simulink model "PSB3_0"  (R2021a)
settings: Solver=VariableStepAuto  StartTime=0.0  StopTime=3000  RelTol=1e-3
values from neighbouring files (symbols this model uses):
  n_channel = 1024    [PSB3_0_script.m]    (also in PSB_FPGAdesign8_script.m)
  parallel_factor = 4    [PSB3_0_script.m]    (also in PSB_FPGAdesign8_script.m)
libraries: xbsIndex_r4 x1051, xrbsSSR_Library x154, dspsrcs4 x26
(part 4 of 8)

== system PSB3_0/Overflow Detector add_re_1 ==
  rst : Inport
  A : Inport  Port=2
  B : Inport  Port=3
  S : Inport  Port=4
  Constant17 : xbsIndex_r4/Constant  const=1  gui_display_data_type=Boolean  arith_type=Boolean  n_bits=16  bin_pt=14  preci_type=Single  exp_width=8  frac_width=24  explicit_period=on  period=1  equ=P=C  opselect=C  inp2=PCIN>>17  opr=+  inp1=P  carry=CIN  dbl_ovrd=off  block_type=constant
  Convert : xbsIndex_r4/Convert  gui_display_data_type=Boolean  arith_type=Boolean  n_bits=16  bin_pt=14  float_type=Single  exp_bits=8  fraction_bits=24  quantization=Truncate  overflow=Wrap  en=off  latency=1  pipeline=off  dbl_ovrd=off  block_type=convert
  Expression : xbsIndex_r4/Expression  expression=(A & B & ~S) | (~A & ~B & S)  align_bp=off  en=off  latency=1  precision=User Defined  arith_type=Unsigned  n_bits=1  bin_pt=0  dbl_ovrd=off  block_type=expr
  Register : xbsIndex_r4/Register  init=0  rst=on  en=on  dbl_ovrd=off  block_type=register
  Vector Delay : xrbsSSR_Library/Vector Delay  sg_latency=2  infoeditControl=Selection of Reset will increase slice count due to use of real FFs and instead of SRLs  en=off  vectorize_en=off  rst=off  reg_retiming=off  block_type=delay_ssr  dbl_ovrd=off  sg_ssr=16  sg_ssr_prev=16  sg_ssr_name=vect_delay
      settings: SourceProductName=Xilinx SSR Blockset
  Vector Delay1 : xrbsSSR_Library/Vector Delay  sg_latency=2  infoeditControl=Selection of Reset will increase slice count due to use of real FFs and instead of SRLs  en=off  vectorize_en=off  rst=off  reg_retiming=off  block_type=delay_ssr  dbl_ovrd=off  sg_ssr=16  sg_ssr_prev=16  sg_ssr_name=vect_delay
      settings: SourceProductName=Xilinx SSR Blockset
  Vector Slice : xrbsSSR_Library/Vector Slice  nbits=1  sg_ssr=16  sg_ssr_prev=16  boolean_output=on  mode=Upper Bit Location + Width  bit1=0  base1=MSB of Input  bit0=0  base0=LSB of Input  dbl_ovrd=off  block_type=slice_ssr  sg_ssr_name=vect_slice
      settings: SourceProductName=Xilinx SSR Blockset  infoedit="The Vector Slice block supports input of vector types. Extracts a given range of bits from each sample of input vector and presents it at the output.  The output type is ordinarily unsigned with binary point at zero, but can be Boolean when the slice is one bit wide.<br><br>Hardware notes: In hardware this block costs nothing."
  Vector Slice1 : xrbsSSR_Library/Vector Slice  nbits=1  sg_ssr=16  sg_ssr_prev=16  boolean_output=on  mode=Upper Bit Location + Width  bit1=0  base1=MSB of Input  bit0=0  base0=LSB of Input  dbl_ovrd=off  block_type=slice_ssr  sg_ssr_name=vect_slice
      settings: SourceProductName=Xilinx SSR Blockset  infoedit="The Vector Slice block supports input of vector types. Extracts a given range of bits from each sample of input vector and presents it at the output.  The output type is ordinarily unsigned with binary point at zero, but can be Boolean when the slice is one bit wide.<br><br>Hardware notes: In hardware this block costs nothing."
  Vector Slice2 : xrbsSSR_Library/Vector Slice  nbits=1  sg_ssr=16  sg_ssr_prev=16  boolean_output=on  mode=Upper Bit Location + Width  bit1=0  base1=MSB of Input  bit0=0  base0=LSB of Input  dbl_ovrd=off  block_type=slice_ssr  sg_ssr_name=vect_slice
      settings: SourceProductName=Xilinx SSR Blockset  infoedit="The Vector Slice block supports input of vector types. Extracts a given range of bits from each sample of input vector and presents it at the output.  The output type is ordinarily unsigned with binary point at zero, but can be Boolean when the slice is one bit wide.<br><br>Hardware notes: In hardware this block costs nothing."
  Vector to Scalar : xrbsSSR_Library/Vector2Scalar  sg_ssr=16  sg_ssr_prev=16  sg_ssr_name=vect_Vector2Scalar  block_type=vector2scalar_ssr
      settings: SourceProductName=Xilinx SSR Blockset
  Vector to Scalar1 : xrbsSSR_Library/Vector2Scalar  sg_ssr=16  sg_ssr_prev=16  sg_ssr_name=vect_Vector2Scalar  block_type=vector2scalar_ssr
      settings: SourceProductName=Xilinx SSR Blockset
  Vector to Scalar2 : xrbsSSR_Library/Vector2Scalar  sg_ssr=16  sg_ssr_prev=16  sg_ssr_name=vect_Vector2Scalar  block_type=vector2scalar_ssr
      settings: SourceProductName=Xilinx SSR Blockset
  ov : Outport
  wires:
  Register/1 -> ov/1
  A/1 -> Vector Slice/1
  rst/1 -> Register/2
  Constant17/1 -> Register/1
  B/1 -> Vector Slice1/1
  S/1 -> Vector Slice2/1
  Vector Slice/1 -> Vector Delay/1
  Vector Slice1/1 -> Vector Delay1/1
  Vector Delay/1 -> Vector to Scalar/1
  Vector Delay1/1 -> Vector to Scalar1/1
  Vector Slice2/1 -> Vector to Scalar2/1
  Vector to Scalar/1 -> Expression/1
  Vector to Scalar1/1 -> Expression/2
  Vector to Scalar2/1 -> Expression/3
  Expression/1 -> Convert/1
  Convert/1 -> Register/3

== system PSB3_0/Overflow Detector add_re_2 ==
  rst : Inport
  A : Inport  Port=2
  B : Inport  Port=3
  S : Inport  Port=4
  Constant17 : xbsIndex_r4/Constant  const=1  gui_display_data_type=Boolean  arith_type=Boolean  n_bits=16  bin_pt=14  preci_type=Single  exp_width=8  frac_width=24  explicit_period=on  period=1  equ=P=C  opselect=C  inp2=PCIN>>17  opr=+  inp1=P  carry=CIN  dbl_ovrd=off  block_type=constant
  Convert : xbsIndex_r4/Convert  gui_display_data_type=Boolean  arith_type=Boolean  n_bits=16  bin_pt=14  float_type=Single  exp_bits=8  fraction_bits=24  quantization=Truncate  overflow=Wrap  en=off  latency=1  pipeline=off  dbl_ovrd=off  block_type=convert
  Expression : xbsIndex_r4/Expression  expression=(A & B & ~S) | (~A & ~B & S)  align_bp=off  en=off  latency=1  precision=User Defined  arith_type=Unsigned  n_bits=1  bin_pt=0  dbl_ovrd=off  block_type=expr
  Register : xbsIndex_r4/Register  init=0  rst=on  en=on  dbl_ovrd=off  block_type=register
  Vector Delay : xrbsSSR_Library/Vector Delay  sg_latency=2  infoeditControl=Selection of Reset will increase slice count due to use of real FFs and instead of SRLs  en=off  vectorize_en=off  rst=off  reg_retiming=off  block_type=delay_ssr  dbl_ovrd=off  sg_ssr=16  sg_ssr_prev=16  sg_ssr_name=vect_delay
      settings: SourceProductName=Xilinx SSR Blockset
  Vector Delay1 : xrbsSSR_Library/Vector Delay  sg_latency=2  infoeditControl=Selection of Reset will increase slice count due to use of real FFs and instead of SRLs  en=off  vectorize_en=off  rst=off  reg_retiming=off  block_type=delay_ssr  dbl_ovrd=off  sg_ssr=16  sg_ssr_prev=16  sg_ssr_name=vect_delay
      settings: SourceProductName=Xilinx SSR Blockset
  Vector Slice : xrbsSSR_Library/Vector Slice  nbits=1  sg_ssr=16  sg_ssr_prev=16  boolean_output=on  mode=Upper Bit Location + Width  bit1=0  base1=MSB of Input  bit0=0  base0=LSB of Input  dbl_ovrd=off  block_type=slice_ssr  sg_ssr_name=vect_slice
      settings: SourceProductName=Xilinx SSR Blockset  infoedit="The Vector Slice block supports input of vector types. Extracts a given range of bits from each sample of input vector and presents it at the output.  The output type is ordinarily unsigned with binary point at zero, but can be Boolean when the slice is one bit wide.<br><br>Hardware notes: In hardware this block costs nothing."
  Vector Slice1 : xrbsSSR_Library/Vector Slice  nbits=1  sg_ssr=16  sg_ssr_prev=16  boolean_output=on  mode=Upper Bit Location + Width  bit1=0  base1=MSB of Input  bit0=0  base0=LSB of Input  dbl_ovrd=off  block_type=slice_ssr  sg_ssr_name=vect_slice
      settings: SourceProductName=Xilinx SSR Blockset  infoedit="The Vector Slice block supports input of vector types. Extracts a given range of bits from each sample of input vector and presents it at the output.  The output type is ordinarily unsigned with binary point at zero, but can be Boolean when the slice is one bit wide.<br><br>Hardware notes: In hardware this block costs nothing."
  Vector Slice2 : xrbsSSR_Library/Vector Slice  nbits=1  sg_ssr=16  sg_ssr_prev=16  boolean_output=on  mode=Upper Bit Location + Width  bit1=0  base1=MSB of Input  bit0=0  base0=LSB of Input  dbl_ovrd=off  block_type=slice_ssr  sg_ssr_name=vect_slice
      settings: SourceProductName=Xilinx SSR Blockset  infoedit="The Vector Slice block supports input of vector types. Extracts a given range of bits from each sample of input vector and presents it at the output.  The output type is ordinarily unsigned with binary point at zero, but can be Boolean when the slice is one bit wide.<br><br>Hardware notes: In hardware this block costs nothing."
  Vector to Scalar : xrbsSSR_Library/Vector2Scalar  sg_ssr=16  sg_ssr_prev=16  sg_ssr_name=vect_Vector2Scalar  block_type=vector2scalar_ssr
      settings: SourceProductName=Xilinx SSR Blockset
  Vector to Scalar1 : xrbsSSR_Library/Vector2Scalar  sg_ssr=16  sg_ssr_prev=16  sg_ssr_name=vect_Vector2Scalar  block_type=vector2scalar_ssr
      settings: SourceProductName=Xilinx SSR Blockset
  Vector to Scalar2 : xrbsSSR_Library/Vector2Scalar  sg_ssr=16  sg_ssr_prev=16  sg_ssr_name=vect_Vector2Scalar  block_type=vector2scalar_ssr
      settings: SourceProductName=Xilinx SSR Blockset
  ov : Outport
  wires:
  Register/1 -> ov/1
  A/1 -> Vector Slice/1
  rst/1 -> Register/2
  Constant17/1 -> Register/1
  B/1 -> Vector Slice1/1
  S/1 -> Vector Slice2/1
  Vector Slice/1 -> Vector Delay/1
  Vector Slice1/1 -> Vector Delay1/1
  Vector Delay/1 -> Vector to Scalar/1
  Vector Delay1/1 -> Vector to Scalar1/1
  Vector Slice2/1 -> Vector to Scalar2/1
  Vector to Scalar/1 -> Expression/1
  Vector to Scalar1/1 -> Expression/2
  Vector to Scalar2/1 -> Expression/3
  Expression/1 -> Convert/1
  Convert/1 -> Register/3

== system PSB3_0/Overflow Detector add_re_3 ==
  rst : Inport
  A : Inport  Port=2
  B : Inport  Port=3
  S : Inport  Port=4
  Constant17 : xbsIndex_r4/Constant  const=1  gui_display_data_type=Boolean  arith_type=Boolean  n_bits=16  bin_pt=14  preci_type=Single  exp_width=8  frac_width=24  explicit_period=on  period=1  equ=P=C  opselect=C  inp2=PCIN>>17  opr=+  inp1=P  carry=CIN  dbl_ovrd=off  block_type=constant
  Convert : xbsIndex_r4/Convert  gui_display_data_type=Boolean  arith_type=Boolean  n_bits=16  bin_pt=14  float_type=Single  exp_bits=8  fraction_bits=24  quantization=Truncate  overflow=Wrap  en=off  latency=1  pipeline=off  dbl_ovrd=off  block_type=convert
  Expression : xbsIndex_r4/Expression  expression=(A & B & ~S) | (~A & ~B & S)  align_bp=off  en=off  latency=1  precision=User Defined  arith_type=Unsigned  n_bits=1  bin_pt=0  dbl_ovrd=off  block_type=expr
  Register : xbsIndex_r4/Register  init=0  rst=on  en=on  dbl_ovrd=off  block_type=register
  Vector Delay : xrbsSSR_Library/Vector Delay  sg_latency=2  infoeditControl=Selection of Reset will increase slice count due to use of real FFs and instead of SRLs  en=off  vectorize_en=off  rst=off  reg_retiming=off  block_type=delay_ssr  dbl_ovrd=off  sg_ssr=16  sg_ssr_prev=16  sg_ssr_name=vect_delay
      settings: SourceProductName=Xilinx SSR Blockset
  Vector Delay1 : xrbsSSR_Library/Vector Delay  sg_latency=2  infoeditControl=Selection of Reset will increase slice count due to use of real FFs and instead of SRLs  en=off  vectorize_en=off  rst=off  reg_retiming=off  block_type=delay_ssr  dbl_ovrd=off  sg_ssr=16  sg_ssr_prev=16  sg_ssr_name=vect_delay
      settings: SourceProductName=Xilinx SSR Blockset
  Vector Slice : xrbsSSR_Library/Vector Slice  nbits=1  sg_ssr=16  sg_ssr_prev=16  boolean_output=on  mode=Upper Bit Location + Width  bit1=0  base1=MSB of Input  bit0=0  base0=LSB of Input  dbl_ovrd=off  block_type=slice_ssr  sg_ssr_name=vect_slice
      settings: SourceProductName=Xilinx SSR Blockset  infoedit="The Vector Slice block supports input of vector types. Extracts a given range of bits from each sample of input vector and presents it at the output.  The output type is ordinarily unsigned with binary point at zero, but can be Boolean when the slice is one bit wide.<br><br>Hardware notes: In hardware this block costs nothing."
  Vector Slice1 : xrbsSSR_Library/Vector Slice  nbits=1  sg_ssr=16  sg_ssr_prev=16  boolean_output=on  mode=Upper Bit Location + Width  bit1=0  base1=MSB of Input  bit0=0  base0=LSB of Input  dbl_ovrd=off  block_type=slice_ssr  sg_ssr_name=vect_slice
      settings: SourceProductName=Xilinx SSR Blockset  infoedit="The Vector Slice block supports input of vector types. Extracts a given range of bits from each sample of input vector and presents it at the output.  The output type is ordinarily unsigned with binary point at zero, but can be Boolean when the slice is one bit wide.<br><br>Hardware notes: In hardware this block costs nothing."
  Vector Slice2 : xrbsSSR_Library/Vector Slice  nbits=1  sg_ssr=16  sg_ssr_prev=16  boolean_output=on  mode=Upper Bit Location + Width  bit1=0  base1=MSB of Input  bit0=0  base0=LSB of Input  dbl_ovrd=off  block_type=slice_ssr  sg_ssr_name=vect_slice
      settings: SourceProductName=Xilinx SSR Blockset  infoedit="The Vector Slice block supports input of vector types. Extracts a given range of bits from each sample of input vector and presents it at the output.  The output type is ordinarily unsigned with binary point at zero, but can be Boolean when the slice is one bit wide.<br><br>Hardware notes: In hardware this block costs nothing."
  Vector to Scalar : xrbsSSR_Library/Vector2Scalar  sg_ssr=16  sg_ssr_prev=16  sg_ssr_name=vect_Vector2Scalar  block_type=vector2scalar_ssr
      settings: SourceProductName=Xilinx SSR Blockset
  Vector to Scalar1 : xrbsSSR_Library/Vector2Scalar  sg_ssr=16  sg_ssr_prev=16  sg_ssr_name=vect_Vector2Scalar  block_type=vector2scalar_ssr
      settings: SourceProductName=Xilinx SSR Blockset
  Vector to Scalar2 : xrbsSSR_Library/Vector2Scalar  sg_ssr=16  sg_ssr_prev=16  sg_ssr_name=vect_Vector2Scalar  block_type=vector2scalar_ssr
      settings: SourceProductName=Xilinx SSR Blockset
  ov : Outport
  wires:
  Register/1 -> ov/1
  A/1 -> Vector Slice/1
  rst/1 -> Register/2
  Constant17/1 -> Register/1
  B/1 -> Vector Slice1/1
  S/1 -> Vector Slice2/1
  Vector Slice/1 -> Vector Delay/1
  Vector Slice1/1 -> Vector Delay1/1
  Vector Delay/1 -> Vector to Scalar/1
  Vector Delay1/1 -> Vector to Scalar1/1
  Vector Slice2/1 -> Vector to Scalar2/1
  Vector to Scalar/1 -> Expression/1
  Vector to Scalar1/1 -> Expression/2
  Vector to Scalar2/1 -> Expression/3
  Expression/1 -> Convert/1
  Convert/1 -> Register/3

== system PSB3_0/Overflow Detector add_re_4 ==
  rst : Inport
  A : Inport  Port=2
  B : Inport  Port=3
  S : Inport  Port=4
  Constant17 : xbsIndex_r4/Constant  const=1  gui_display_data_type=Boolean  arith_type=Boolean  n_bits=16  bin_pt=14  preci_type=Single  exp_width=8  frac_width=24  explicit_period=on  period=1  equ=P=C  opselect=C  inp2=PCIN>>17  opr=+  inp1=P  carry=CIN  dbl_ovrd=off  block_type=constant
  Convert : xbsIndex_r4/Convert  gui_display_data_type=Boolean  arith_type=Boolean  n_bits=16  bin_pt=14  float_type=Single  exp_bits=8  fraction_bits=24  quantization=Truncate  overflow=Wrap  en=off  latency=1  pipeline=off  dbl_ovrd=off  block_type=convert
  Expression : xbsIndex_r4/Expression  expression=(A & B & ~S) | (~A & ~B & S)  align_bp=off  en=off  latency=1  precision=User Defined  arith_type=Unsigned  n_bits=1  bin_pt=0  dbl_ovrd=off  block_type=expr
  Register : xbsIndex_r4/Register  init=0  rst=on  en=on  dbl_ovrd=off  block_type=register
  Vector Delay : xrbsSSR_Library/Vector Delay  sg_latency=2  infoeditControl=Selection of Reset will increase slice count due to use of real FFs and instead of SRLs  en=off  vectorize_en=off  rst=off  reg_retiming=off  block_type=delay_ssr  dbl_ovrd=off  sg_ssr=16  sg_ssr_prev=16  sg_ssr_name=vect_delay
      settings: SourceProductName=Xilinx SSR Blockset
  Vector Delay1 : xrbsSSR_Library/Vector Delay  sg_latency=2  infoeditControl=Selection of Reset will increase slice count due to use of real FFs and instead of SRLs  en=off  vectorize_en=off  rst=off  reg_retiming=off  block_type=delay_ssr  dbl_ovrd=off  sg_ssr=16  sg_ssr_prev=16  sg_ssr_name=vect_delay
      settings: SourceProductName=Xilinx SSR Blockset
  Vector Slice : xrbsSSR_Library/Vector Slice  nbits=1  sg_ssr=16  sg_ssr_prev=16  boolean_output=on  mode=Upper Bit Location + Width  bit1=0  base1=MSB of Input  bit0=0  base0=LSB of Input  dbl_ovrd=off  block_type=slice_ssr  sg_ssr_name=vect_slice
      settings: SourceProductName=Xilinx SSR Blockset  infoedit="The Vector Slice block supports input of vector types. Extracts a given range of bits from each sample of input vector and presents it at the output.  The output type is ordinarily unsigned with binary point at zero, but can be Boolean when the slice is one bit wide.<br><br>Hardware notes: In hardware this block costs nothing."
  Vector Slice1 : xrbsSSR_Library/Vector Slice  nbits=1  sg_ssr=16  sg_ssr_prev=16  boolean_output=on  mode=Upper Bit Location + Width  bit1=0  base1=MSB of Input  bit0=0  base0=LSB of Input  dbl_ovrd=off  block_type=slice_ssr  sg_ssr_name=vect_slice
      settings: SourceProductName=Xilinx SSR Blockset  infoedit="The Vector Slice block supports input of vector types. Extracts a given range of bits from each sample of input vector and presents it at the output.  The output type is ordinarily unsigned with binary point at zero, but can be Boolean when the slice is one bit wide.<br><br>Hardware notes: In hardware this block costs nothing."
  Vector Slice2 : xrbsSSR_Library/Vector Slice  nbits=1  sg_ssr=16  sg_ssr_prev=16  boolean_output=on  mode=Upper Bit Location + Width  bit1=0  base1=MSB of Input  bit0=0  base0=LSB of Input  dbl_ovrd=off  block_type=slice_ssr  sg_ssr_name=vect_slice
      settings: SourceProductName=Xilinx SSR Blockset  infoedit="The Vector Slice block supports input of vector types. Extracts a given range of bits from each sample of input vector and presents it at the output.  The output type is ordinarily unsigned with binary point at zero, but can be Boolean when the slice is one bit wide.<br><br>Hardware notes: In hardware this block costs nothing."
  Vector to Scalar : xrbsSSR_Library/Vector2Scalar  sg_ssr=16  sg_ssr_prev=16  sg_ssr_name=vect_Vector2Scalar  block_type=vector2scalar_ssr
      settings: SourceProductName=Xilinx SSR Blockset
  Vector to Scalar1 : xrbsSSR_Library/Vector2Scalar  sg_ssr=16  sg_ssr_prev=16  sg_ssr_name=vect_Vector2Scalar  block_type=vector2scalar_ssr
      settings: SourceProductName=Xilinx SSR Blockset
  Vector to Scalar2 : xrbsSSR_Library/Vector2Scalar  sg_ssr=16  sg_ssr_prev=16  sg_ssr_name=vect_Vector2Scalar  block_type=vector2scalar_ssr
      settings: SourceProductName=Xilinx SSR Blockset
  ov : Outport
  wires:
  Register/1 -> ov/1
  A/1 -> Vector Slice/1
  rst/1 -> Register/2
  Constant17/1 -> Register/1
  B/1 -> Vector Slice1/1
  S/1 -> Vector Slice2/1
  Vector Slice/1 -> Vector Delay/1
  Vector Slice1/1 -> Vector Delay1/1
  Vector Delay/1 -> Vector to Scalar/1
  Vector Delay1/1 -> Vector to Scalar1/1
  Vector Slice2/1 -> Vector to Scalar2/1
  Vector to Scalar/1 -> Expression/1
  Vector to Scalar1/1 -> Expression/2
  Vector to Scalar2/1 -> Expression/3
  Expression/1 -> Convert/1
  Convert/1 -> Register/3

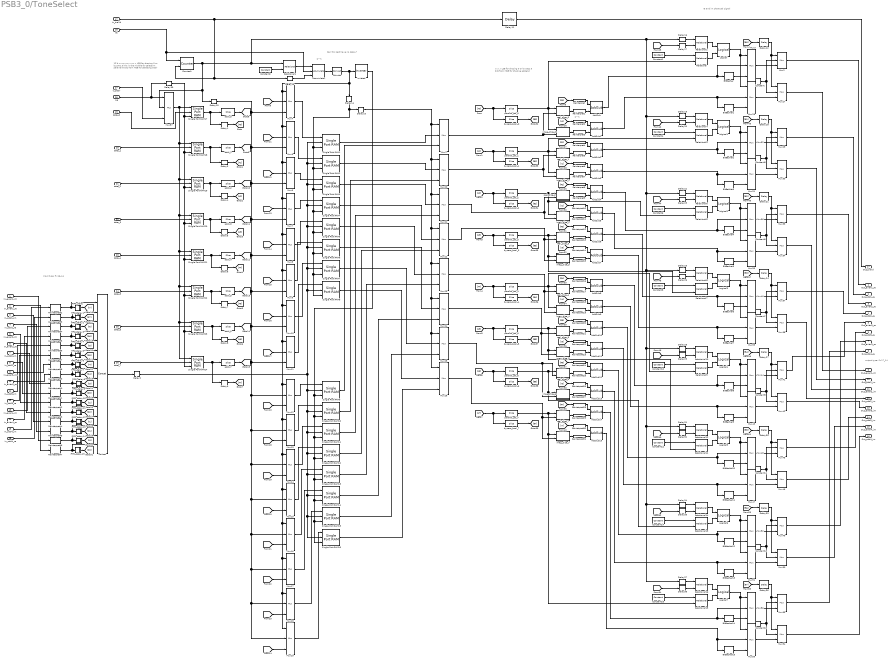
== system PSB3_0/ToneSelect ==
  note: Can this cast have no delay?
  note: Z^-1
  note: input type: fix16_14
  note: output type: fix17_14
  note: xxx,x
      | LSB for chosing 0 or bypass
      | 3 bits from MSB for chosing addend
  note: re and im share sel signal
  note: Z^-1
  note: 12'b xxxxxxxx,xxx,x
      | LSB for chosing 0 or bypass
      | 3 bits in the middle for selecting parallel
      | 8 bits from MSB for selecting addr
  In_even1_im : Inport
  In_even1_re : Inport  Port=2
  In_odd1_im : Inport  Port=3
  In_odd1_re : Inport  Port=4
  In_even2_im : Inport  Port=5
  In_even2_re : Inport  Port=6
  In_odd2_im : Inport  Port=7
  In_odd2_re : Inport  Port=8
  In_even3_im : Inport  Port=9
  In_even3_re : Inport  Port=10
  In_odd3_im : Inport  Port=11
  In_odd3_re : Inport  Port=12
  In_even4_im : Inport  Port=13
  In_even4_re : Inport  Port=14
  In_odd4_im : Inport  Port=15
  In_odd4_re : Inport  Port=16
  In_tvalid : Inport  Port=17
  rst : Inport  Port=18
  data_0 : Inport  Port=19
  data_1 : Inport  Port=20
  data_2 : Inport  Port=21
  data_3 : Inport  Port=22
  data_4 : Inport  Port=23
  data_5 : Inport  Port=24
  data_6 : Inport  Port=25
  data_7 : Inport  Port=26
  w_addr : Inport  Port=27
  we : Inport  Port=28
  Accumulator : xbsIndex_r4/Accumulator  operation=Add  n_bits=1  overflow=Wrap  scale=1  rst=on  hasbypass=off  infoeditControl=reset for floating point data type must be asserted for a minimum of 2 cycles  en=on  latency=1  msb_inp=1  msb=1  lsb=1  use_behavioral_HDL=on  implementation=Fabric  dbl_ovrd=off  block_type=accum
  AddSub{,1..15} (16 alike) : xbsIndex_r4/AddSub  mode=Addition  use_carryin=off  use_carryout=off  en=off  latency=2  precision=User Defined  arith_type="Signed  (2's comp)"  n_bits=17  bin_pt=14  quantization=Truncate  overflow=Flag as error  use_behavioral_HDL=off  hw_selection=Fabric  pipelined=off  dbl_ovrd=off  block_type=addsub
  BitBasher{,1..15} (16 alike) : xbsIndex_r4/BitBasher  bitexpr=o={i[16],i[16:1]}  display_expr=off  sr_1=o  arith_type1="Signed  (2's comp)"  bin_pt1=14  sr_2=2  arith_type2=Unsigned  bin_pt2=0  sr_3=3  arith_type3=Unsigned  bin_pt3=0  sr_4=4  arith_type4=Unsigned  bin_pt4=0  dbl_ovrd=off  block_type=bitbasher
  Concat : xbsIndex_r4/Concat  num_inputs=16  dbl_ovrd=off  block_type=concat
  Constant{,3,5,7,9,11,13,15} (8 alike) : xbsIndex_r4/Constant  const=0  gui_display_data_type=Fixed-point  arith_type=Signed (2's comp)  n_bits=17  bin_pt=14  preci_type=Single  exp_width=8  frac_width=24  explicit_period=on  period=1  equ=P=C  opselect=C  inp2=PCIN>>17  opr=+  inp1=P  carry=CIN  dbl_ovrd=off  block_type=constant
  Constant1 : xbsIndex_r4/Constant  const=0  gui_display_data_type=Fixed-point  arith_type=Unsigned  n_bits=3  bin_pt=0  preci_type=Single  exp_width=8  frac_width=24  explicit_period=on  period=1  equ=P=C  opselect=C  inp2=PCIN>>17  opr=+  inp1=P  carry=CIN  dbl_ovrd=off  block_type=constant
  Constant10 : xbsIndex_r4/Constant  const=4  gui_display_data_type=Fixed-point  arith_type=Unsigned  n_bits=3  bin_pt=0  preci_type=Single  exp_width=8  frac_width=24  explicit_period=on  period=1  equ=P=C  opselect=C  inp2=PCIN>>17  opr=+  inp1=P  carry=CIN  dbl_ovrd=off  block_type=constant
  Constant12 : xbsIndex_r4/Constant  const=5  gui_display_data_type=Fixed-point  arith_type=Unsigned  n_bits=3  bin_pt=0  preci_type=Single  exp_width=8  frac_width=24  explicit_period=on  period=1  equ=P=C  opselect=C  inp2=PCIN>>17  opr=+  inp1=P  carry=CIN  dbl_ovrd=off  block_type=constant
  Constant14 : xbsIndex_r4/Constant  const=6  gui_display_data_type=Fixed-point  arith_type=Unsigned  n_bits=3  bin_pt=0  preci_type=Single  exp_width=8  frac_width=24  explicit_period=on  period=1  equ=P=C  opselect=C  inp2=PCIN>>17  opr=+  inp1=P  carry=CIN  dbl_ovrd=off  block_type=constant
  Constant16 : xbsIndex_r4/Constant  const=7  gui_display_data_type=Fixed-point  arith_type=Unsigned  n_bits=3  bin_pt=0  preci_type=Single  exp_width=8  frac_width=24  explicit_period=on  period=1  equ=P=C  opselect=C  inp2=PCIN>>17  opr=+  inp1=P  carry=CIN  dbl_ovrd=off  block_type=constant
  Constant2 : xbsIndex_r4/Constant  const=0  gui_display_data_type=Fixed-point  arith_type=Unsigned  n_bits=8  bin_pt=0  preci_type=Single  exp_width=8  frac_width=24  explicit_period=on  period=1  equ=P=C  opselect=C  inp2=PCIN>>17  opr=+  inp1=P  carry=CIN  dbl_ovrd=off  block_type=constant
  Constant4 : xbsIndex_r4/Constant  const=1  gui_display_data_type=Fixed-point  arith_type=Unsigned  n_bits=3  bin_pt=0  preci_type=Single  exp_width=8  frac_width=24  explicit_period=on  period=1  equ=P=C  opselect=C  inp2=PCIN>>17  opr=+  inp1=P  carry=CIN  dbl_ovrd=off  block_type=constant
  Constant6 : xbsIndex_r4/Constant  const=2  gui_display_data_type=Fixed-point  arith_type=Unsigned  n_bits=3  bin_pt=0  preci_type=Single  exp_width=8  frac_width=24  explicit_period=on  period=1  equ=P=C  opselect=C  inp2=PCIN>>17  opr=+  inp1=P  carry=CIN  dbl_ovrd=off  block_type=constant
  Constant8 : xbsIndex_r4/Constant  const=3  gui_display_data_type=Fixed-point  arith_type=Unsigned  n_bits=3  bin_pt=0  preci_type=Single  exp_width=8  frac_width=24  explicit_period=on  period=1  equ=P=C  opselect=C  inp2=PCIN>>17  opr=+  inp1=P  carry=CIN  dbl_ovrd=off  block_type=constant
  Convert : xbsIndex_r4/Convert  gui_display_data_type=Boolean  arith_type=Boolean  n_bits=16  bin_pt=14  float_type=Single  exp_bits=8  fraction_bits=24  quantization=Truncate  overflow=Wrap  en=off  latency=0  pipeline=off  dbl_ovrd=off  block_type=convert
  Counter1 : xbsIndex_r4/Counter  cnt_type=Free Running  cnt_to=Inf  operation=Up  start_count=0  cnt_by_val=1  arith_type=Unsigned  n_bits=8  bin_pt=0  load_pin=off  rst=on  en=on  explicit_period=on  period=1  use_behavioral_HDL=off  implementation=Fabric  dbl_ovrd=off  block_type=counter
  Delay{1..9,17,20,23,26,29,32,35,38} (17 alike) : xbsIndex_r4/Delay  rst=off  infoeditControl=Selection of Reset will increase slice count due to use of real FFs and instead of SRLs  en=off  latency=3  reg_retiming=off  dbl_ovrd=off  block_type=delay
  Delay10 : xbsIndex_r4/Delay  rst=off  infoeditControl=Selection of Reset will increase slice count due to use of real FFs and instead of SRLs  en=off  latency=1  reg_retiming=off  dbl_ovrd=off  block_type=delay
  Delay11 : xbsIndex_r4/Delay  rst=off  infoeditControl=Selection of Reset will increase slice count due to use of real FFs and instead of SRLs  en=off  latency=10+256  reg_retiming=off  dbl_ovrd=off  block_type=delay
  Delay{12,18,21,24,27,30,33,36} (8 alike) : xbsIndex_r4/Delay  rst=off  infoeditControl=Selection of Reset will increase slice count due to use of real FFs and instead of SRLs  en=off  latency=4  reg_retiming=off  dbl_ovrd=off  block_type=delay
  Delay{13,16,19,22,25,28,31,34,37} (9 alike) : xbsIndex_r4/Delay  rst=off  infoeditControl=Selection of Reset will increase slice count due to use of real FFs and instead of SRLs  en=off  latency=5  reg_retiming=off  dbl_ovrd=off  block_type=delay
  Delay14 : xbsIndex_r4/Delay  rst=off  infoeditControl=Selection of Reset will increase slice count due to use of real FFs and instead of SRLs  en=off  latency=1  reg_retiming=off  dbl_ovrd=off  block_type=delay
  Delay15 : xbsIndex_r4/Delay  rst=off  infoeditControl=Selection of Reset will increase slice count due to use of real FFs and instead of SRLs  en=off  latency=2  reg_retiming=off  dbl_ovrd=off  block_type=delay
  Delay39 : xbsIndex_r4/Delay  rst=off  infoeditControl=Selection of Reset will increase slice count due to use of real FFs and instead of SRLs  en=off  latency=1  reg_retiming=off  dbl_ovrd=off  block_type=delay
  FIFO_delay : Subsystem
  FIFO_delay1 : Subsystem
  FIFO_delay10 : Subsystem
  FIFO_delay11 : Subsystem
  FIFO_delay12 : Subsystem
  FIFO_delay13 : Subsystem
  FIFO_delay14 : Subsystem
  FIFO_delay15 : Subsystem
  FIFO_delay2 : Subsystem
  FIFO_delay3 : Subsystem
  FIFO_delay4 : Subsystem
  FIFO_delay5 : Subsystem
  FIFO_delay6 : Subsystem
  FIFO_delay7 : Subsystem
  FIFO_delay8 : Subsystem
  FIFO_delay9 : Subsystem
  Inverter : xbsIndex_r4/Inverter  en=off  latency=1  dbl_ovrd=off  block_type=inv
  Logical{,1..7} (8 alike) : xbsIndex_r4/Logical  logical_function=AND  inputs=2  en=off  latency=1  precision=Full  arith_type=Unsigned  n_bits=16  bin_pt=0  align_bp=on  dbl_ovrd=off  block_type=logical
  Mux{1..57} (57 alike) : xbsIndex_r4/Mux  inputs=2  en=off  latency=1  precision=Full  arith_type="Signed  (2's comp)"  n_bits=17  bin_pt=14  quantization=Truncate  overflow=Flag as error  dbl_ovrd=off  block_type=mux
  Reinterpret{,1..31} (32 alike) : xbsIndex_r4/Reinterpret  force_arith_type=on  arith_type="Signed  (2's comp)"  force_bin_pt=on  bin_pt=14  block_type=reinterpret
  Reinterpret{32..47} (16 alike) : xbsIndex_r4/Reinterpret  force_arith_type=on  arith_type=Unsigned  force_bin_pt=on  bin_pt=0  block_type=reinterpret
  Relational{,2..16} (16 alike) : xbsIndex_r4/Relational  mode=a=b  op_type=Bool  en=off  latency=2  dbl_ovrd=off  block_type=relational
  Relational1 : xbsIndex_r4/Relational  mode=a=b  op_type=Ufix  en=off  latency=1  dbl_ovrd=off  block_type=relational
  Single Port RAM{1..16} (16 alike) : xbsIndex_r4/Single Port RAM  depth=256  initVector=0  distributed_mem=Block RAM  write_mode=Read After Write  rst=off  init_reg=0  en=off  optimize_latency=off  latency=1  optimize=Area  dbl_ovrd=off  simulation_type=fast_sim  block_type=spram
  Single Port RAM17 : xbsIndex_r4/Single Port RAM  depth=256  initVector=toneMap_0  distributed_mem=Block RAM  write_mode=Read After Write  rst=off  init_reg=0  en=off  optimize_latency=off  latency=1  optimize=Area  dbl_ovrd=off  simulation_type=fast_sim  block_type=spram
  Single Port RAM18 : xbsIndex_r4/Single Port RAM  depth=256  initVector=toneMap_1  distributed_mem=Block RAM  write_mode=Read After Write  rst=off  init_reg=0  en=off  optimize_latency=off  latency=1  optimize=Area  dbl_ovrd=off  simulation_type=fast_sim  block_type=spram
  Single Port RAM19 : xbsIndex_r4/Single Port RAM  depth=256  initVector=toneMap_2  distributed_mem=Block RAM  write_mode=Read After Write  rst=off  init_reg=0  en=off  optimize_latency=off  latency=1  optimize=Area  dbl_ovrd=off  simulation_type=fast_sim  block_type=spram
  Single Port RAM20 : xbsIndex_r4/Single Port RAM  depth=256  initVector=toneMap_3  distributed_mem=Block RAM  write_mode=Read After Write  rst=off  init_reg=0  en=off  optimize_latency=off  latency=1  optimize=Area  dbl_ovrd=off  simulation_type=fast_sim  block_type=spram
  Single Port RAM21 : xbsIndex_r4/Single Port RAM  depth=256  initVector=toneMap_4  distributed_mem=Block RAM  write_mode=Read After Write  rst=off  init_reg=0  en=off  optimize_latency=off  latency=1  optimize=Area  dbl_ovrd=off  simulation_type=fast_sim  block_type=spram
  Single Port RAM22 : xbsIndex_r4/Single Port RAM  depth=256  initVector=toneMap_5  distributed_mem=Block RAM  write_mode=Read After Write  rst=off  init_reg=0  en=off  optimize_latency=off  latency=1  optimize=Area  dbl_ovrd=off  simulation_type=fast_sim  block_type=spram
  Single Port RAM23 : xbsIndex_r4/Single Port RAM  depth=256  initVector=toneMap_6  distributed_mem=Block RAM  write_mode=Read After Write  rst=off  init_reg=0  en=off  optimize_latency=off  latency=1  optimize=Area  dbl_ovrd=off  simulation_type=fast_sim  block_type=spram
  Single Port RAM24 : xbsIndex_r4/Single Port RAM  depth=256  initVector=toneMap_7  distributed_mem=Block RAM  write_mode=Read After Write  rst=off  init_reg=0  en=off  optimize_latency=off  latency=1  optimize=Area  dbl_ovrd=off  simulation_type=fast_sim  block_type=spram
  addr_{0..7} (8 alike) : xbsIndex_r4/Slice  nbits=8  boolean_output=off  mode=Lower Bit Location + Width  bit1=0  base1=MSB of Input  bit0=4  base0=LSB of Input  dbl_ovrd=off  block_type=slice
  bypass_bool_{0..7} (8 alike) : xbsIndex_r4/Slice  nbits=1  boolean_output=on  mode=Lower Bit Location + Width  bit1=0  base1=MSB of Input  bit0=0  base0=LSB of Input  dbl_ovrd=off  block_type=slice
  imag_slice_0 : Subsystem
  imag_slice_1 : Subsystem
  imag_slice_2 : Subsystem
  imag_slice_3 : Subsystem
  imag_slice_4 : Subsystem
  imag_slice_5 : Subsystem
  imag_slice_6 : Subsystem
  imag_slice_7 : Subsystem
  parallel_sel_{0..7} (8 alike) : xbsIndex_r4/Slice  nbits=3  boolean_output=off  mode=Lower Bit Location + Width  bit1=0  base1=MSB of Input  bit0=1  base0=LSB of Input  dbl_ovrd=off  block_type=slice
  real_slice_0 : Subsystem
  real_slice_1 : Subsystem
  real_slice_2 : Subsystem
  real_slice_3 : Subsystem
  real_slice_4 : Subsystem
  real_slice_5 : Subsystem
  real_slice_6 : Subsystem
  real_slice_7 : Subsystem
  Out_even1_re : Outport
  Out_odd1_re : Outport  Port=2
  Out_even2_re : Outport  Port=3
  Out_odd2_re : Outport  Port=4
  Out_even3_re : Outport  Port=5
  Out_odd3_re : Outport  Port=6
  Out_even4_re : Outport  Port=7
  Out_odd4_re : Outport  Port=8
  Out_even1_im : Outport  Port=9
  Out_odd1_im : Outport  Port=10
  Out_even2_im : Outport  Port=11
  Out_odd2_im : Outport  Port=12
  Out_even3_im : Outport  Port=13
  Out_odd3_im : Outport  Port=14
  Out_even4_im : Outport  Port=15
  Out_odd4_im : Outport  Port=16
  Out_tvalid : Outport  Port=17
  wires:
  rst/1 -> Accumulator/2, Counter1/1
  In_tvalid/1 -> Delay11/1, Delay13/1, Counter1/2
  Delay11/1 -> Out_tvalid/1
  Concat/1 -> Delay2/1
  Constant2/1 -> Relational1/2
  Relational1/1 -> Accumulator/1
  Delay13/1 -> Accumulator/3
  Accumulator/1 -> Convert/1
  Inverter/1 -> Single Port RAM9/3, Single Port RAM10/3, Single Port RAM11/3, Single Port RAM12/3, Single Port RAM13/3, Single Port RAM14/3, Single Port RAM15/3, Single Port RAM16/3
  Mux4/1 -> Single Port RAM1/1
  Single Port RAM17/1 -> Delay1/1, addr_0/1
  Delay14/1 -> Single Port RAM1/3, Single Port RAM2/3, Single Port RAM8/3, Single Port RAM7/3, Single Port RAM6/3, Single Port RAM5/3, Single Port RAM4/3, Single Port RAM3/3, Delay10/1
  Delay15/1 -> Mux4/3, Mux5/3, Mux9/3, Mux11/3, Mux12/2, Mux13/2, Mux14/2, Mux15/2, Mux16/2, Mux17/2, Mux19/2, Mux18/2, Mux10/3, Mux8/3, Mux7/3, Mux6/3
  Single Port RAM18/1 -> addr_1/1, Delay3/1
  Mux5/1 -> Single Port RAM2/1
  Single Port RAM19/1 -> addr_2/1, Delay4/1
  Mux6/1 -> Single Port RAM3/1
  Single Port RAM20/1 -> addr_3/1, Delay5/1
  Single Port RAM21/1 -> addr_4/1, Delay6/1
  Mux7/1 -> Single Port RAM4/1
  Mux8/1 -> Single Port RAM5/1
  Single Port RAM22/1 -> addr_5/1, Delay7/1
  Mux9/1 -> Single Port RAM6/1
  Single Port RAM23/1 -> addr_6/1, Delay8/1
  Mux10/1 -> Single Port RAM7/1
  Single Port RAM24/1 -> Delay9/1, addr_7/1
  Mux11/1 -> Single Port RAM8/1
  Mux12/1 -> Single Port RAM9/1
  Mux13/1 -> Single Port RAM10/1
  Mux14/1 -> Single Port RAM11/1
  Mux15/1 -> Single Port RAM12/1
  Mux16/1 -> Single Port RAM13/1
  Mux17/1 -> Single Port RAM14/1
  Mux18/1 -> Single Port RAM15/1
  Mux19/1 -> Single Port RAM16/1
  [A0] -> bypass_bool_0/1, parallel_sel_0/1
  [A1] -> bypass_bool_1/1, parallel_sel_1/1
  [A2] -> bypass_bool_2/1, parallel_sel_2/1
  [A3] -> bypass_bool_3/1, parallel_sel_3/1
  [A4] -> bypass_bool_4/1, parallel_sel_4/1
  [A5] -> bypass_bool_5/1, parallel_sel_5/1
  [A6] -> bypass_bool_6/1, parallel_sel_6/1
  [A7] -> bypass_bool_7/1, parallel_sel_7/1
  real_slice_0/1(output) -> Reinterpret1/1
  Delay1/1 -> [A0]
  Delay3/1 -> [A1]
  Delay4/1 -> [A2]
  Delay5/1 -> [A3]
  Delay6/1 -> [A4]
  Delay7/1 -> [A5]
  Delay8/1 -> [A6]
  Delay9/1 -> [A7]
  parallel_sel_1/1 -> Relational3/2, imag_slice_1/1(sel), real_slice_1/1(sel)
  Single Port RAM1/1 -> Mux1/2
  Single Port RAM2/1 -> Mux20/2
  Delay2/1 -> Single Port RAM6/2, Single Port RAM4/2, Single Port RAM3/2, Single Port RAM2/2, Single Port RAM1/2, Single Port RAM5/2, Single Port RAM7/2, Single Port RAM8/2, Single Port RAM16/2, Single Port RAM15/2, Single Port RAM14/2, Single Port RAM13/2, Single Port RAM12/2, Single Port RAM11/2, Single Port RAM10/2, Single Port RAM9/2
  Delay10/1 -> Mux26/1, Mux25/1, Mux24/1, Mux23/1, Mux22/1, Mux21/1, Mux20/1, Mux1/1
  Single Port RAM3/1 -> Mux21/2
  Single Port RAM4/1 -> Mux22/2
  Single Port RAM5/1 -> Mux23/2
  Single Port RAM6/1 -> Mux24/2
  Single Port RAM7/1 -> Mux25/2
  Single Port RAM8/1 -> Mux26/2
  Single Port RAM9/1 -> Mux1/3
  Single Port RAM10/1 -> Mux20/3
  Single Port RAM11/1 -> Mux21/3
  Single Port RAM12/1 -> Mux22/3
  Single Port RAM13/1 -> Mux23/3
  Single Port RAM14/1 -> Mux24/3
  Single Port RAM15/1 -> Mux25/3
  Single Port RAM16/1 -> Mux26/3
  addr_0/1 -> [addr0]
  addr_1/1 -> [addr1]
  addr_2/1 -> [addr2]
  addr_3/1 -> [addr3]
  addr_4/1 -> [addr4]
  addr_5/1 -> [addr5]
  addr_6/1 -> [addr6]
  addr_7/1 -> [addr7]
  parallel_sel_2/1 -> Relational5/2, imag_slice_2/1(sel), real_slice_2/1(sel)
  parallel_sel_3/1 -> Relational7/2, imag_slice_3/1(sel), real_slice_3/1(sel)
  parallel_sel_4/1 -> imag_slice_4/1(sel), Relational9/2, real_slice_4/1(sel)
  parallel_sel_5/1 -> Relational11/2, imag_slice_5/1(sel), real_slice_5/1(sel)
  parallel_sel_6/1 -> imag_slice_6/1(sel), Relational13/2, real_slice_6/1(sel)
  parallel_sel_7/1 -> Relational15/2, imag_slice_7/1(sel), real_slice_7/1(sel)
  Mux1/1 -> real_slice_0/2(input), imag_slice_0/2(input)
  Mux20/1 -> imag_slice_1/2(input), real_slice_1/2(input)
  Mux21/1 -> imag_slice_2/2(input), real_slice_2/2(input)
  bypass_bool_0/1 -> [B0]
  Mux22/1 -> imag_slice_3/2(input), real_slice_3/2(input)
  Mux23/1 -> imag_slice_4/2(input), real_slice_4/2(input)
  Mux24/1 -> imag_slice_5/2(input), real_slice_5/2(input)
  Mux25/1 -> imag_slice_6/2(input), real_slice_6/2(input)
  Mux26/1 -> imag_slice_7/2(input), real_slice_7/2(input)
  bypass_bool_1/1 -> [B1]
  bypass_bool_2/1 -> [B2]
  bypass_bool_3/1 -> [B3]
  bypass_bool_4/1 -> [B4]
  bypass_bool_5/1 -> [B5]
  bypass_bool_6/1 -> [B6]
  bypass_bool_7/1 -> [B7]
  imag_slice_7/1(output) -> Reinterpret31/1
  real_slice_7/1(output) -> Reinterpret29/1
  imag_slice_6/1(output) -> Reinterpret27/1
  real_slice_6/1(output) -> Reinterpret25/1
  imag_slice_5/1(output) -> Reinterpret23/1
  real_slice_5/1(output) -> Reinterpret21/1
  imag_slice_4/1(output) -> Reinterpret19/1
  real_slice_4/1(output) -> Reinterpret17/1
  imag_slice_3/1(output) -> Reinterpret15/1
  real_slice_3/1(output) -> Reinterpret13/1
  imag_slice_2/1(output) -> Reinterpret11/1
  real_slice_2/1(output) -> Reinterpret9/1
  imag_slice_1/1(output) -> Reinterpret7/1
  real_slice_1/1(output) -> Reinterpret5/1
  imag_slice_0/1(output) -> Reinterpret3/1
  In_even1_re/1 -> Reinterpret47/1
  In_even1_im/1 -> Reinterpret46/1
  In_odd1_re/1 -> Reinterpret45/1
  In_odd1_im/1 -> Reinterpret44/1
  In_even2_re/1 -> Reinterpret43/1
  In_even2_im/1 -> Reinterpret42/1
  In_odd2_re/1 -> Reinterpret41/1
  In_odd2_im/1 -> Reinterpret40/1
  In_even3_re/1 -> Reinterpret39/1
  In_even3_im/1 -> Reinterpret38/1
  In_odd3_re/1 -> Reinterpret37/1
  In_odd3_im/1 -> Reinterpret36/1
  In_even4_re/1 -> Reinterpret35/1
  In_even4_im/1 -> Reinterpret34/1
  In_odd4_re/1 -> Reinterpret33/1
  In_odd4_im/1 -> Reinterpret32/1
  Counter1/1 -> Relational1/1, Delay16/1, Delay37/1, Delay34/1, Delay31/1, Delay28/1, Delay25/1, Delay22/1, Delay19/1, Delay15/1, Mux57/2
  Mux3/1 -> Mux2/3
  Constant1/1 -> Relational/1
  AddSub/1 -> BitBasher/1, Mux3/2
  Relational/1 -> Logical/2
  Relational2/1 -> Logical/1
  parallel_sel_0/1 -> real_slice_0/1(sel), Relational/2, imag_slice_0/1(sel)
  Delay17/1 -> Relational2/2
  BitBasher/1 -> Mux3/3
  [B0] -> Delay12/1
  [addr0] -> Delay17/1
  Delay16/1 -> Relational2/1
  Logical/1 -> Mux28/1, Mux3/1
  Mux28/1 -> Mux27/3
  Delay12/1 -> Mux2/1, Mux27/1
  BitBasher1/1 -> Mux28/3
  Constant/1 -> Mux27/2, Mux2/2
  AddSub1/1 -> BitBasher1/1, Mux28/2
  [B1] -> Delay18/1
  AddSub3/1 -> BitBasher3/1, Mux31/2
  AddSub2/1 -> BitBasher2/1, Mux32/2
  Delay20/1 -> Relational4/2
  [addr1] -> Delay20/1
  Relational3/1 -> Logical1/2
  Constant4/1 -> Relational3/1
  BitBasher2/1 -> Mux32/3
  Delay19/1 -> Relational4/1
  Relational4/1 -> Logical1/1
  Delay18/1 -> Mux29/1, Mux30/1
  Logical1/1 -> Mux31/1, Mux32/1
  Mux32/1 -> Mux29/3
  Constant3/1 -> Mux30/2, Mux29/2
  BitBasher3/1 -> Mux31/3
  Mux31/1 -> Mux30/3
  [B2] -> Delay21/1
  AddSub5/1 -> BitBasher5/1, Mux35/2
  AddSub4/1 -> BitBasher4/1, Mux36/2
  Delay23/1 -> Relational6/2
  [addr2] -> Delay23/1
  Relational5/1 -> Logical2/2
  Constant6/1 -> Relational5/1
  BitBasher4/1 -> Mux36/3
  Delay22/1 -> Relational6/1
  Relational6/1 -> Logical2/1
  Delay21/1 -> Mux33/1, Mux34/1
  Logical2/1 -> Mux35/1, Mux36/1
  Mux36/1 -> Mux33/3
  Constant5/1 -> Mux34/2, Mux33/2
  BitBasher5/1 -> Mux35/3
  Mux35/1 -> Mux34/3
  [B3] -> Delay24/1
  Delay26/1 -> Relational8/2
  [addr3] -> Delay26/1
  Relational7/1 -> Logical3/2
  Constant8/1 -> Relational7/1
  BitBasher6/1 -> Mux40/3
  Delay25/1 -> Relational8/1
  Relational8/1 -> Logical3/1
  Delay24/1 -> Mux37/1, Mux38/1
  Logical3/1 -> Mux39/1, Mux40/1
  Mux40/1 -> Mux37/3
  Constant7/1 -> Mux38/2, Mux37/2
  BitBasher7/1 -> Mux39/3
  Mux39/1 -> Mux38/3
  [B4] -> Delay27/1
  AddSub9/1 -> BitBasher9/1, Mux43/2
  AddSub8/1 -> BitBasher8/1, Mux44/2
  Delay29/1 -> Relational10/2
  [addr4] -> Delay29/1
  Relational9/1 -> Logical4/2
  Constant10/1 -> Relational9/1
  BitBasher8/1 -> Mux44/3
  Delay28/1 -> Relational10/1
  Relational10/1 -> Logical4/1
  Delay27/1 -> Mux41/1, Mux42/1
  Logical4/1 -> Mux43/1, Mux44/1
  Mux44/1 -> Mux41/3
  Constant9/1 -> Mux42/2, Mux41/2
  BitBasher9/1 -> Mux43/3
  Mux43/1 -> Mux42/3
  [B5] -> Delay30/1
  AddSub11/1 -> BitBasher11/1, Mux47/2
  AddSub10/1 -> BitBasher10/1, Mux48/2
  Delay32/1 -> Relational12/2
  [addr5] -> Delay32/1
  Relational11/1 -> Logical5/2
  Constant12/1 -> Relational11/1
  BitBasher10/1 -> Mux48/3
  Delay31/1 -> Relational12/1
  Relational12/1 -> Logical5/1
  Delay30/1 -> Mux45/1, Mux46/1
  Logical5/1 -> Mux47/1, Mux48/1
  Mux48/1 -> Mux45/3
  Constant11/1 -> Mux46/2, Mux45/2
  BitBasher11/1 -> Mux47/3
  Mux47/1 -> Mux46/3
  [B6] -> Delay33/1
  AddSub13/1 -> BitBasher13/1, Mux51/2
  AddSub12/1 -> BitBasher12/1, Mux52/2
  Delay35/1 -> Relational14/2
  [addr6] -> Delay35/1
  Relational13/1 -> Logical6/2
  Constant14/1 -> Relational13/1
  BitBasher12/1 -> Mux52/3
  Delay34/1 -> Relational14/1
  Relational14/1 -> Logical6/1
  Delay33/1 -> Mux49/1, Mux50/1
  Logical6/1 -> Mux51/1, Mux52/1
  Mux52/1 -> Mux49/3
  Constant13/1 -> Mux50/2, Mux49/2
  BitBasher13/1 -> Mux51/3
  Mux51/1 -> Mux50/3
  [B7] -> Delay36/1
  AddSub15/1 -> BitBasher15/1, Mux55/2
  AddSub14/1 -> BitBasher14/1, Mux56/2
  Delay38/1 -> Relational16/2
  [addr7] -> Delay38/1
  Relational15/1 -> Logical7/2
  Constant16/1 -> Relational15/1
  BitBasher14/1 -> Mux56/3
  Delay37/1 -> Relational16/1
  Relational16/1 -> Logical7/1
  Delay36/1 -> Mux53/1, Mux54/1
  Logical7/1 -> Mux55/1, Mux56/1
  Mux56/1 -> Mux53/3
  Constant15/1 -> Mux54/2, Mux53/2
  BitBasher15/1 -> Mux55/3
  Mux55/1 -> Mux54/3
  AddSub6/1 -> BitBasher6/1, Mux40/2
  AddSub7/1 -> BitBasher7/1, Mux39/2
  Mux2/1 -> Out_even1_re/1
  Mux27/1 -> Out_even1_im/1
  Mux29/1 -> Out_odd1_re/1
  Mux30/1 -> Out_odd1_im/1
  Mux33/1 -> Out_even2_re/1
  Mux34/1 -> Out_even2_im/1
  Mux37/1 -> Out_odd2_re/1
  Mux38/1 -> Out_odd2_im/1
  Mux41/1 -> Out_even3_re/1
  Mux42/1 -> Out_even3_im/1
  Mux45/1 -> Out_odd3_re/1
  Mux46/1 -> Out_odd3_im/1
  Mux49/1 -> Out_even4_re/1
  Mux50/1 -> Out_even4_im/1
  Mux53/1 -> Out_odd4_re/1
  Mux54/1 -> Out_odd4_im/1
  we/1 -> Mux57/1, Delay39/1
  w_addr/1 -> Mux57/3
  Mux57/1 -> Single Port RAM17/1, Single Port RAM24/1, Single Port RAM23/1, Single Port RAM22/1, Single Port RAM21/1, Single Port RAM20/1, Single Port RAM19/1, Single Port RAM18/1
  Delay39/1 -> Single Port RAM24/3, Single Port RAM23/3, Single Port RAM22/3, Single Port RAM21/3, Single Port RAM20/3, Single Port RAM19/3, Single Port RAM18/3, Single Port RAM17/3
  data_0/1 -> Single Port RAM17/2
  data_1/1 -> Single Port RAM18/2
  data_2/1 -> Single Port RAM19/2
  data_3/1 -> Single Port RAM20/2
  data_4/1 -> Single Port RAM21/2
  data_5/1 -> Single Port RAM22/2
  data_6/1 -> Single Port RAM23/2
  data_7/1 -> Single Port RAM24/2
  Reinterpret1/1 -> AddSub/2
  [R0] -> Reinterpret/1
  Reinterpret/1 -> AddSub/1
  [I0] -> Reinterpret2/1
  Reinterpret2/1 -> AddSub1/1
  Reinterpret3/1 -> AddSub1/2
  [R1] -> Reinterpret4/1
  Reinterpret4/1 -> AddSub2/1
  Reinterpret5/1 -> AddSub2/2
  Reinterpret6/1 -> AddSub3/1
  [I1] -> Reinterpret6/1
  Reinterpret7/1 -> AddSub3/2
  [R2] -> Reinterpret8/1
  Reinterpret8/1 -> AddSub4/1
  Reinterpret9/1 -> AddSub4/2
  Reinterpret10/1 -> AddSub5/1
  [I2] -> Reinterpret10/1
  Reinterpret11/1 -> AddSub5/2
  [R3] -> Reinterpret12/1
  Reinterpret12/1 -> AddSub6/1
  Reinterpret13/1 -> AddSub6/2
  [I3] -> Reinterpret14/1
  Reinterpret14/1 -> AddSub7/1
  Reinterpret15/1 -> AddSub7/2
  [R4] -> Reinterpret16/1
  Reinterpret16/1 -> AddSub8/1
  Reinterpret17/1 -> AddSub8/2
  [I4] -> Reinterpret18/1
  Reinterpret18/1 -> AddSub9/1
  Reinterpret19/1 -> AddSub9/2
  [R5] -> Reinterpret20/1
  Reinterpret20/1 -> AddSub10/1
  Reinterpret21/1 -> AddSub10/2
  Reinterpret22/1 -> AddSub11/1
  [I5] -> Reinterpret22/1
  Reinterpret23/1 -> AddSub11/2
  Reinterpret24/1 -> AddSub12/1
  [R6] -> Reinterpret24/1
  Reinterpret25/1 -> AddSub12/2
  [I6] -> Reinterpret26/1
  Reinterpret26/1 -> AddSub13/1
  Reinterpret27/1 -> AddSub13/2
  [R7] -> Reinterpret28/1
  Reinterpret28/1 -> AddSub14/1
  Reinterpret29/1 -> AddSub14/2
  [I7] -> Reinterpret30/1
  Reinterpret30/1 -> AddSub15/1
  Reinterpret31/1 -> AddSub15/2
  Reinterpret32/1 -> FIFO_delay/1(In1), Concat/1
  Reinterpret33/1 -> FIFO_delay1/1(In1), Concat/2
  Reinterpret34/1 -> FIFO_delay2/1(In1), Concat/3
  Reinterpret35/1 -> FIFO_delay3/1(In1), Concat/4
  Reinterpret36/1 -> FIFO_delay4/1(In1), Concat/5
  Reinterpret37/1 -> FIFO_delay5/1(In1), Concat/6
  Reinterpret38/1 -> FIFO_delay6/1(In1), Concat/7
  Reinterpret39/1 -> Concat/8, FIFO_delay7/1(In1)
  Reinterpret40/1 -> FIFO_delay8/1(In1), Concat/9
  Reinterpret41/1 -> FIFO_delay9/1(In1), Concat/10
  Reinterpret42/1 -> FIFO_delay10/1(In1), Concat/11
  Reinterpret43/1 -> FIFO_delay11/1(In1), Concat/12
  Reinterpret44/1 -> FIFO_delay12/1(In1), Concat/13
  Reinterpret45/1 -> FIFO_delay13/1(In1), Concat/14
  Reinterpret46/1 -> FIFO_delay14/1(In1), Concat/15
  Reinterpret47/1 -> FIFO_delay15/1(In1), Concat/16
  Convert/1 -> Delay14/1, Mux14/1, Mux15/1, Mux16/1, Mux17/1, Mux18/1, Mux19/1, Mux13/1, Mux12/1, Mux11/1, Mux10/1, Mux9/1, Mux8/1, Mux7/1, Mux6/1, Mux5/1, Mux4/1, Inverter/1
  FIFO_delay/1(Out1) -> [I7]
  FIFO_delay1/1(Out1) -> [R7]
  FIFO_delay2/1(Out1) -> [I6]
  FIFO_delay3/1(Out1) -> [R6]
  FIFO_delay4/1(Out1) -> [I5]
  FIFO_delay5/1(Out1) -> [R5]
  FIFO_delay6/1(Out1) -> [I4]
  FIFO_delay7/1(Out1) -> [R4]
  FIFO_delay15/1(Out1) -> [R0]
  FIFO_delay8/1(Out1) -> [I3]
  FIFO_delay9/1(Out1) -> [R3]
  FIFO_delay10/1(Out1) -> [I2]
  FIFO_delay11/1(Out1) -> [R2]
  FIFO_delay12/1(Out1) -> [I1]
  FIFO_delay13/1(Out1) -> [R1]
  FIFO_delay14/1(Out1) -> [I0]
  [addr0] -> Mux4/2
  [addr1] -> Mux5/2
  [addr2] -> Mux6/2
  [addr3] -> Mux7/2
  [addr4] -> Mux8/2
  [addr5] -> Mux9/2
  [addr6] -> Mux10/2
  [addr7] -> Mux11/2
  [addr0] -> Mux12/3
  [addr1] -> Mux13/3
  [addr2] -> Mux14/3
  [addr3] -> Mux15/3
  [addr4] -> Mux16/3
  [addr5] -> Mux17/3
  [addr6] -> Mux18/3
  [addr7] -> Mux19/3

== system PSB3_0/delayCounter ==
  note: Counter that is enabled after the first rising edge1, and disabled after the first rising edge2. Need to calibrate the initial value of counter before getting desired delay value.
  edge1 : Inport
  edge2 : Inport  Port=2
  Counter1 : xbsIndex_r4/Counter  cnt_type=Free Running  cnt_to=Inf  operation=Up  start_count=0  cnt_by_val=1  arith_type=Unsigned  n_bits=12  bin_pt=0  load_pin=off  rst=off  en=on  explicit_period=on  period=1  use_behavioral_HDL=off  implementation=DSP48  dbl_ovrd=off  block_type=counter
  Logical : xbsIndex_r4/Logical  logical_function=XOR  inputs=2  en=off  latency=1  precision=User Defined  arith_type=Boolean  n_bits=1  bin_pt=0  align_bp=on  dbl_ovrd=off  block_type=logical
  Register1 : xbsIndex_r4/Register  init=0  rst=off  en=on  dbl_ovrd=off  block_type=register
  Register2 : xbsIndex_r4/Register  init=0  rst=off  en=on  dbl_ovrd=off  block_type=register
  const1 : xbsIndex_r4/Constant  const=1  gui_display_data_type=Boolean  arith_type=Boolean  n_bits=18  bin_pt=16  preci_type=Single  exp_width=8  frac_width=24  explicit_period=on  period=1  equ=P=C  opselect=C  inp2=PCIN>>17  opr=+  inp1=P  carry=CIN  dbl_ovrd=off  block_type=constant
  delay : Outport
  wires:
  Counter1/1 -> delay/1
  Register2/1 -> Logical/2
  Logical/1 -> Counter1/1
  const1/1 -> Register1/1, Register2/1
  Register1/1 -> Logical/1
  edge2/1 -> Register2/2
  edge1/1 -> Register1/2
